simulink model "Photothermal"  (Simulink 10.3)
settings: Solver=VariableStepAuto  StartTime=0.0  StopTime=86400  RelTol=1e-3  AbsTol=1e-3
PreLoadFcn:
  | pipe_area = 0.01; % m^2
  | furnace_temperature = 1500; % degC
  | boiler_liquid_level = 0.7; % 1
  | condenser_liquid_level = 0.2;
  | preheat_condenser_liquid_level = 0.2; % 1
undefined symbols (not defined in the file or in its folder): sigbuilder_block
libraries: fl_lib x42, nesl_utility x11, RankineCycle_lib x5, pid_lib x2
(part 1 of 3)
Description:
  | Rankine Cycle (Steam Turbine)
CloseFcn:
  | try,close(h1_ssc_rankine_cycle),end
  | clear h1_ssc_rankine_cycle
  | try,close(h2_ssc_rankine_cycle),end
  | clear h2_ssc_rankine_cycle
  | try,close(h3_ssc_rankine_cycle),end
  | clear h3_ssc_rankine_cycle
  | 
  | clear simlog_ssc_rankine_cycle tout
  | clear pipe_area furnace_temperature boiler_liquid_level condenser_liquid_level preheat_condenser_liquid_level
settings Model: Creator=The MathWorks, Inc.  LastModifiedBy=ss  MultithreadedSim=on
settings SolverCC: AutoScaleAbsTol=off  MaxConsecutiveMinStep=2
settings DataIOCC: LimitDataPoints=on  MaxDataPoints=10000  SaveFormat=Dataset  SignalLoggingSaveFormat=Dataset
settings OptimizationCC: ExpressionDepthLimit=128  LifeSpan=auto
settings DebuggingCC: UnderspecifiedInitializationDetection=Simplified  MergeDetectMultiDrivingBlocksExec=error  FcnCallInpInsideContextMsg=error  StateNameClashWarn=none  PregeneratedLibrarySubsystemCodeDiagnostic=none  SFUnexpectedBacktrackingDiag=error  SFNoUnconditionalDefaultTransitionDiag=error  SFExecutionAtInitializationDiag=warning
settings HardwareCC: ProdBitPerPointer=64  ProdBitPerSizeT=64  ProdBitPerPtrDiffT=64  ProdLargestAtomicFloat=Float  ProdIntDivRoundTo=Zero  ProdEndianess=LittleEndian  ProdWordSize=64  ProdHWDeviceType=Intel->x86-64 (Windows64)
settings ModelReferenceCC: PropagateSignalLabelsOutOfModel=on
settings GRTTargetCC: TargetLangStandard=C99 (ISO)  CombineOutputUpdateFcns=on  GRTInterface=off
settings ConfigComp: CovMetricSettings=dwe  CovSaveCumulativeToWorkspaceVar=off  CovSaveSingleToWorkspaceVar=off  CovExternalEMLEnable=on
settings SimscapeCC: SimscapeLogType=all  SimscapeLogSimulationStatistics=on  SimscapeLogName=simlog_ssc_rankine_cycle  SimscapeLogDataHistory=10000

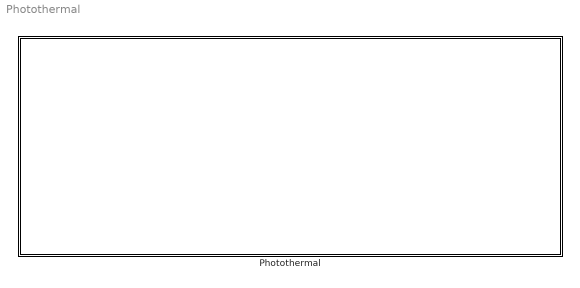
== system Photothermal ==
  Photothermal : Subsystem
